simulink model "base_trans_recv_QPSK"  (R2024b)
settings: Solver=FixedStepDiscrete  StartTime=0.0  StopTime=Param.TotalFrame * Param.FrameTime  RelTol=1e-3
undefined symbols (not defined in the file): Param
libraries: commchan3 x1, commdigbbndpm3 x1
settings Model: Creator=roberto  LastModifiedBy=rober
settings RTWCC: GPUComputeCapability=3.5

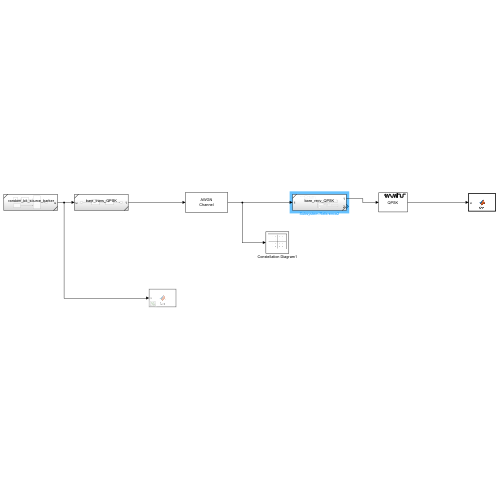
[thumbnail: Simulink's stored preview of the top-level diagram]
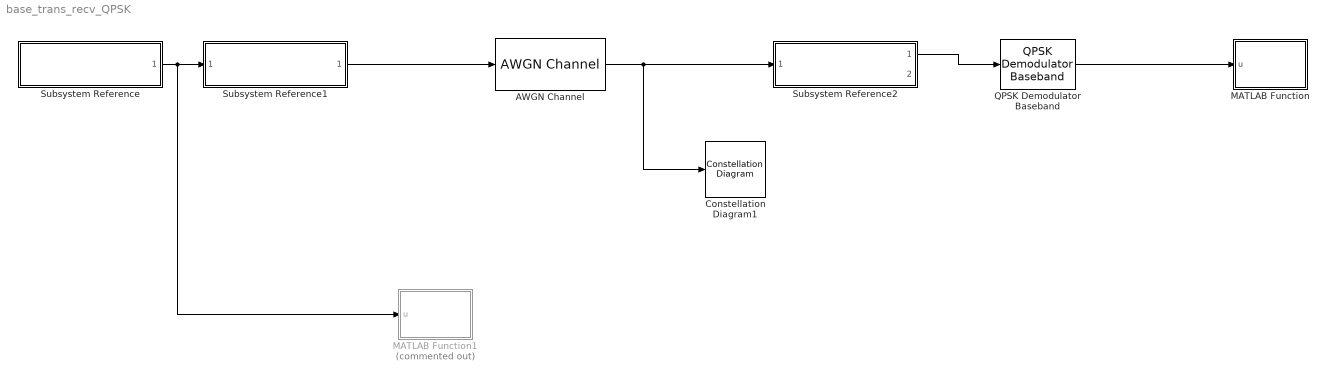
== system base_trans_recv_QPSK ==
  AWGN Channel : commchan3/AWGN Channel  LegacyMode=off  NoiseMethod="Signal to noise ratio  (Eb/No)"  noiseMode="Signal to noise ratio  (SNR)"  EbNo=20  EsNo=10  SNR=20  BitsPerSymbol=log2(Param.ModulationOrder)  SignalPower=1/Param.Interpolation  SamplesPerSymbol=Param.Interpolation  SymbolPeriod=1  VarianceSource=Parameter  Variance=1  RandomStream=Global stream  Seed=67  SimulateUsing=Code generation
  Constellation Diagram1 : ConstellationDiagram  WindowPosition=[753.000000,89.000000,600.000000,600.000000,]  Visible=on  ScopeFrameLocation=window
  MATLAB Function : MATLAB Function  TreatAsAtomicUnit=on
  MATLAB Function1 : MATLAB Function  Commented=on  TreatAsAtomicUnit=on
  QPSK Demodulator Baseband : commdigbbndpm3/QPSK Demodulator Baseband  OutType=Bit  DecType=Hard decision  VarSource=Dialog  Variance=1  Dec=Gray  Ph=pi/4  outDtype1=Inherit via internal rule  outDtype2=Inherit via internal rule  derotateFactorWordLen=16  derotateFactorDataTypeStr=Inherit: Same word length as input  derotateFactorLastDataTypeStr=Inherit: Same word length as input
  Subsystem Reference : Subsystem  ReferencedSubsystem=random_bit_source_barker
  Subsystem Reference1 : Subsystem  ReferencedSubsystem=bare_trans_QPSK
  Subsystem Reference2 : Subsystem  ReferencedSubsystem=bare_recv_QPSK
  wires:
  Subsystem Reference2/1 -> QPSK Demodulator Baseband/1
  QPSK Demodulator Baseband/1 -> MATLAB Function/1(u)
  AWGN Channel/1 -> Constellation Diagram1/1, Subsystem Reference2/1
  Subsystem Reference1/1 -> AWGN Channel/1
  Subsystem Reference/1 -> MATLAB Function1/1(u), Subsystem Reference1/1

== matlab function base_trans_recv_QPSK/MATLAB Function ==
  data: u input
function fcn(u)
fprintf("%s\n", char(u'+ '0'));
end

== matlab function base_trans_recv_QPSK/MATLAB Function1 ==
  data: u input
function fcn(u)
    fprintf("%s\n", char(u'+ '0'));
end
